simulink model "LqrSpeedTest1"  (R2018a)
settings: Solver=VariableStepAuto  StartTime=0.0  StopTime=15  RelTol=1e-3
values from neighbouring files (symbols this model uses):
  A = Gss.A    [TFfinder.m]
  B = Gss.B    [TFfinder.m]
  C = tf(PID*Gm)    [PIDtest1.m]    (also in TFfinder.m = Gss.C)
settings Model: Creator=Yahya  LastModifiedBy=mmbio
settings CodeAppCC: StateflowObjectComments=on

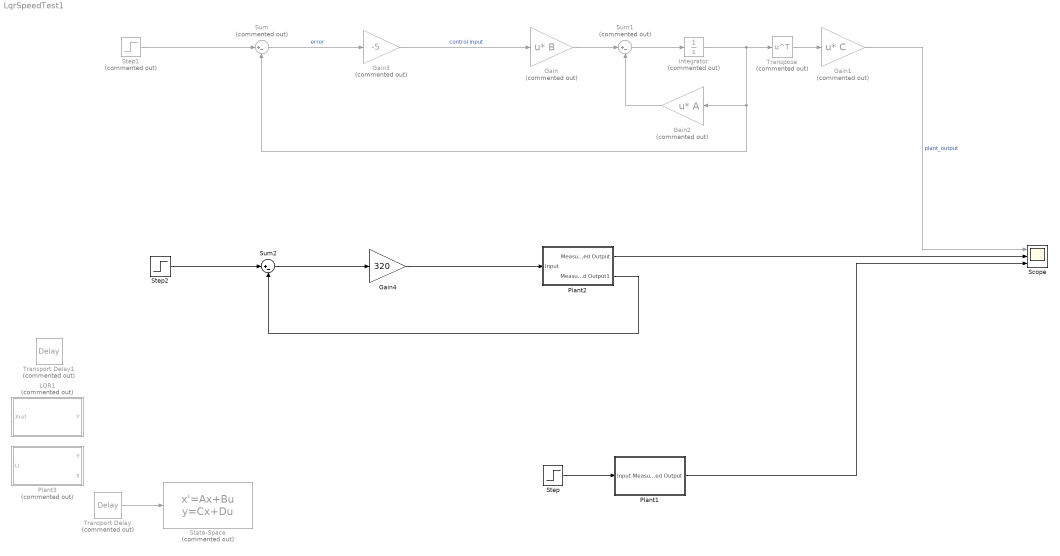
== system LqrSpeedTest1 ==
  Gain : Gain  Commented=on  Gain=B  Multiplication=Matrix(u*K)
  Gain1 : Gain  Commented=on  Gain=C  Multiplication=Matrix(u*K)
  Gain2 : Gain  Commented=on  Gain=A  Multiplication=Matrix(u*K)
  Gain3 : Gain  Commented=on  Gain=-5
  Gain4 : Gain  Gain=320
  Integrator : Integrator  Commented=on
  LQR1 : Subsystem  Commented=on
  Plant1 : Subsystem
  Plant2 : Subsystem
  Plant3 : Subsystem  Commented=on
  Scope : Scope  NumInputPorts=3
  State-Space : StateSpace  Commented=on  A=A  B=B  C=C  D=0  InitialCondition=0
  Step : Step  SampleTime=0
  Step1 : Step  Commented=on  SampleTime=0
  Step2 : Step  SampleTime=0
  Sum : Sum  Commented=on  Inputs=|+-
  Sum1 : Sum  Commented=on  Inputs=|+-
  Sum2 : Sum  Inputs=|+-
  Transport Delay : TransportDelay  Commented=on  DelayTime=0.3
  Transport Delay1 : TransportDelay  Commented=on  DelayTime=0.3
  Transpose : Math  Commented=on  Operator=transpose  SaturateOnIntegerOverflow=on
  wires:
  Sum/1 -> Gain3/1  "error"
  Step/1 -> Plant1/1(Input)
  Integrator/1 -> Transpose/1, Gain2/1, Sum/2
  Gain1/1 -> Scope/1  "plant_output"
  Sum1/1 -> Integrator/1
  Gain2/1 -> Sum1/2
  Gain/1 -> Sum1/1
  Gain3/1 -> Gain/1  "control input"
  Step1/1 -> Sum/1
  Transpose/1 -> Gain1/1
  Gain4/1 -> Plant2/1(Input)
  Plant1/1(Measured Output) -> Scope/3
  Transport Delay/1 -> State-Space/1
  Plant2/1(Measured Output) -> Scope/2
  Step2/1 -> Sum2/1
  Sum2/1 -> Gain4/1
  Plant2/2(Measured Output1) -> Sum2/2

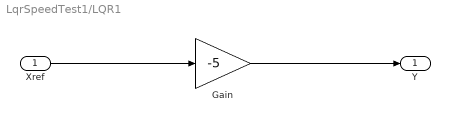
== system LqrSpeedTest1/LQR1 ==
  Xref : Inport
  Gain : Gain  Gain=-5
  Y : Outport
  wires:
  Xref/1 -> Gain/1
  Gain/1 -> Y/1

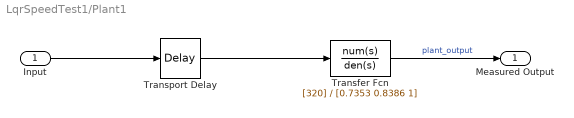
== system LqrSpeedTest1/Plant1 ==
  Input : Inport
  Transfer Fcn : TransferFcn  Numerator=[320]  Denominator=[0.7353 0.8386 1]
  Transport Delay : TransportDelay  DelayTime=0.3
  Measured Output : Outport
  wires:
  Input/1 -> Transport Delay/1
  Transfer Fcn/1 -> Measured Output/1  "plant_output"
  Transport Delay/1 -> Transfer Fcn/1

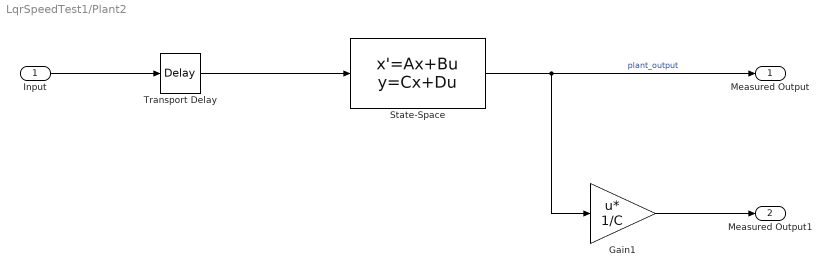
== system LqrSpeedTest1/Plant2 ==
  Input : Inport
  Gain1 : Gain  Gain=1/C  Multiplication=Matrix(u*K)
  State-Space : StateSpace  A=A  B=B  C=C  D=0  InitialCondition=0
  Transport Delay : TransportDelay  DelayTime=0.3
  Measured Output : Outport
  Measured Output1 : Outport  Port=2
  wires:
  Input/1 -> Transport Delay/1
  State-Space/1 -> Gain1/1, Measured Output/1  "plant_output"
  Transport Delay/1 -> State-Space/1
  Gain1/1 -> Measured Output1/1

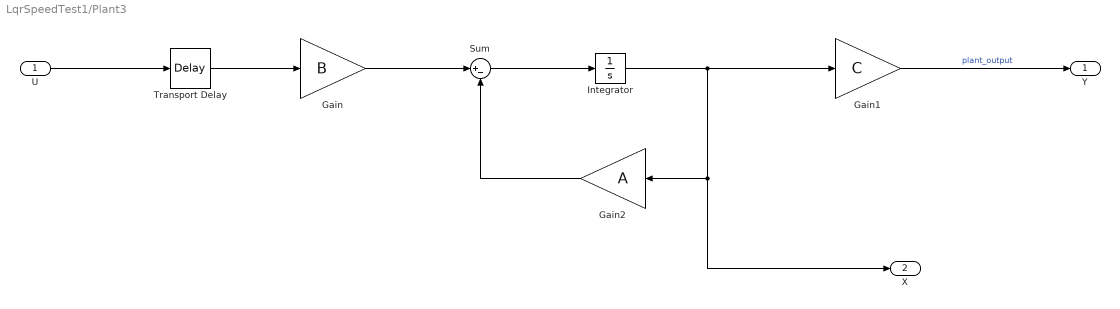
== system LqrSpeedTest1/Plant3 ==
  U : Inport
  Gain : Gain  Gain=B
  Gain1 : Gain  Gain=C
  Gain2 : Gain  Gain=A
  Integrator : Integrator
  Sum : Sum  Inputs=|+-
  Transport Delay : TransportDelay  DelayTime=0.3
  Y : Outport
  X : Outport  Port=2
  wires:
  U/1 -> Transport Delay/1
  Gain1/1 -> Y/1  "plant_output"
  Sum/1 -> Integrator/1
  Gain/1 -> Sum/1
  Integrator/1 -> Gain2/1, X/1, Gain1/1
  Gain2/1 -> Sum/2
  Transport Delay/1 -> Gain/1
